simulink model "blockmodel"  (R2017b)
settings: Solver=VariableStepAuto  StartTime=0.0  StopTime=100.0  RelTol=1e-3
PreLoadFcn:
  | tic
values from neighbouring files (symbols this model uses):
  a = 1    [init.m]
  a_m = -4    [init.m]
  b = 3    [init.m]
  b_m = 4    [init.m]
  x_m_0 = 0    [init.m]
  x_p_0 = 0    [init.m]
CloseFcn:
  | toc
settings Model: Creator=q3  LastModifiedBy=q3

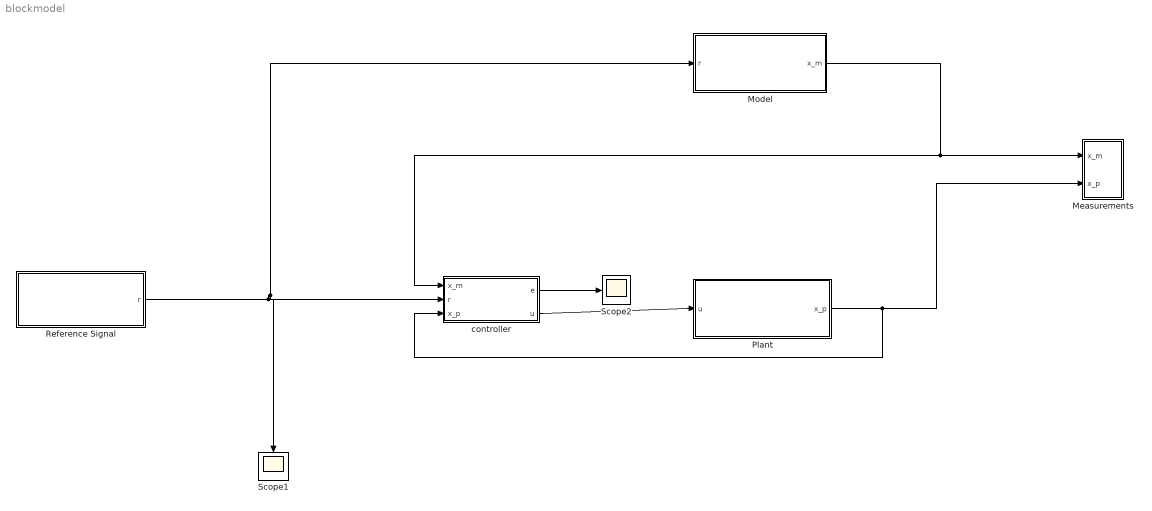
== system blockmodel ==
  Measurements : Subsystem
  Model : Subsystem
  Plant : Subsystem
  Reference Signal : Subsystem
  Scope1 : Scope
  Scope2 : Scope
  controller : Subsystem
  wires:
  controller/2(u) -> Plant/1(u)
  Model/1(x_m) -> controller/1(x_m), Measurements/1(x_m)
  Plant/1(x_p) -> controller/3(x_p), Measurements/2(x_p)
  controller/1(e) -> Scope2/1
  Reference Signal/1(r) -> Model/1(r), controller/2(r), Scope1/1

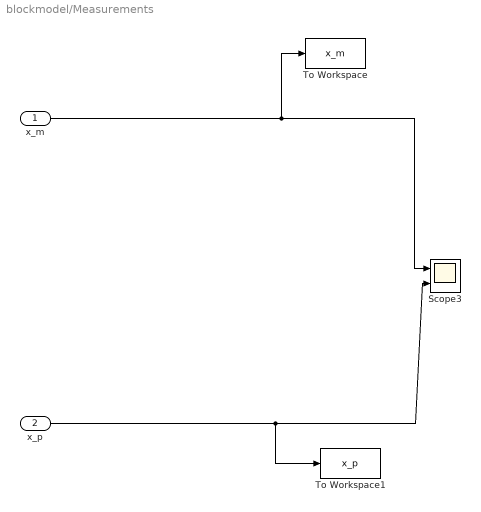
== system blockmodel/Measurements ==
  x_m : Inport
  x_p : Inport  Port=2
  Scope3 : Scope  NumInputPorts=2
  To Workspace : ToWorkspace  VariableName=x_m  SaveFormat=Timeseries  SampleTime=-1
  To Workspace1 : ToWorkspace  VariableName=x_p  SaveFormat=Timeseries  SampleTime=-1
  wires:
  x_p/1 -> Scope3/2, To Workspace1/1
  x_m/1 -> To Workspace/1, Scope3/1

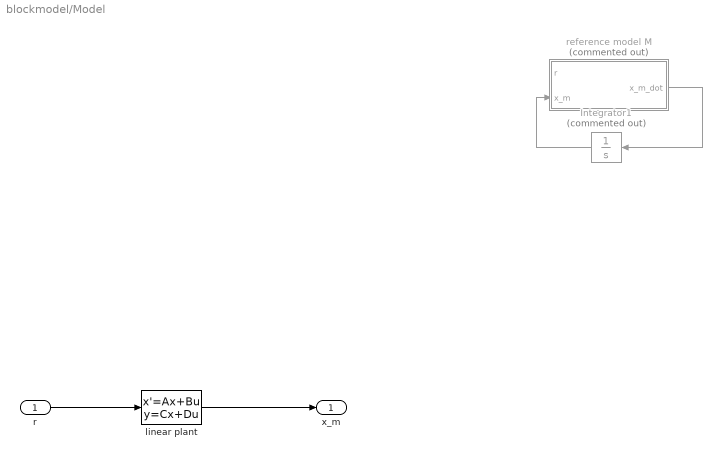
== system blockmodel/Model ==
  r : Inport
  Integrator1 : Integrator  Commented=on  InitialCondition=x_m_0
  linear plant : StateSpace  A=a_m  B=b_m  D=0  InitialCondition=x_m_0
  reference model M : MATLAB Function  Commented=on  TreatAsAtomicUnit=on
  x_m : Outport
  wires:
  reference model M/1(x_m_dot) -> Integrator1/1
  Integrator1/1 -> reference model M/2(x_m)
  r/1 -> linear plant/1
  linear plant/1 -> x_m/1

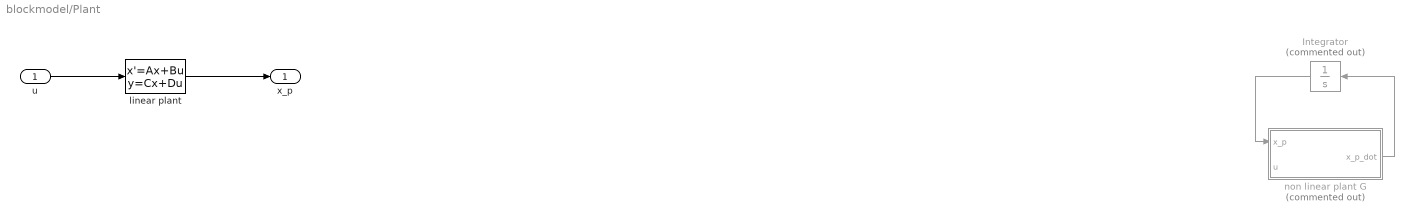
== system blockmodel/Plant ==
  u : Inport
  Integrator : Integrator  Commented=on  InitialCondition=x_p_0
  linear plant : StateSpace  A=a  B=b  D=0  InitialCondition=x_p_0
  non linear plant G : MATLAB Function  Commented=on  TreatAsAtomicUnit=on
  x_p : Outport
  wires:
  Integrator/1 -> non linear plant G/1(x_p)
  non linear plant G/1(x_p_dot) -> Integrator/1
  u/1 -> linear plant/1
  linear plant/1 -> x_p/1

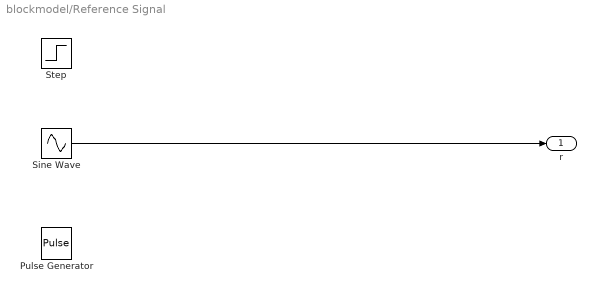
== system blockmodel/Reference Signal ==
  Pulse Generator : DiscretePulseGenerator  PulseType=Time based  Amplitude=4  PulseWidth=5
  Sine Wave : Sin  Amplitude=4  Frequency=4  SampleTime=0
  Step : Step  After=4  SampleTime=0
  r : Outport
  wires:
  Sine Wave/1 -> r/1

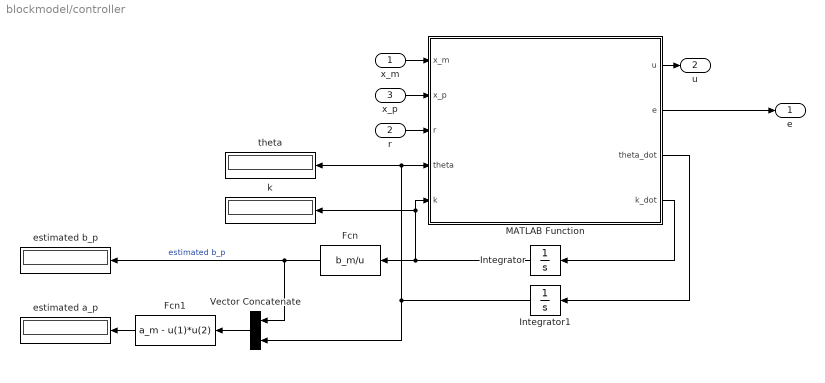
== system blockmodel/controller ==
  x_m : Inport
  r : Inport  Port=2
  x_p : Inport  Port=3
  Fcn : Fcn  Expr=b_m/u
  Fcn1 : Fcn  Expr=a_m - u(1)*u(2)
  Integrator : Integrator
  Integrator1 : Integrator
  MATLAB Function : MATLAB Function  TreatAsAtomicUnit=on
  Vector Concatenate : Concatenate
  estimated a_p : Display
  estimated b_p : Display
  k : Display
  theta : Display
  e : Outport
  u : Outport  Port=2
  wires:
  Integrator1/1 -> Vector Concatenate/2, MATLAB Function/4(theta), theta/1
  MATLAB Function/4(k_dot) -> Integrator/1
  Integrator/1 -> Fcn/1, k/1, MATLAB Function/5(k)
  MATLAB Function/2(e) -> e/1
  x_p/1 -> MATLAB Function/2(x_p)
  MATLAB Function/1(u) -> u/1
  MATLAB Function/3(theta_dot) -> Integrator1/1
  r/1 -> MATLAB Function/3(r)
  x_m/1 -> MATLAB Function/1(x_m)
  Fcn/1 -> Vector Concatenate/1, estimated b_p/1  "estimated b_p"
  Vector Concatenate/1 -> Fcn1/1
  Fcn1/1 -> estimated a_p/1

== matlab function blockmodel/Model/reference model M ==
  data: r input; x_m input; x_m_dot output
function x_m_dot = fcn(r,x_m)

% reference model equation
x_m_dot = -4*x_m + 4*r;

== matlab function blockmodel/controller/MATLAB Function ==
  data: u output; e output; x_m input; theta_dot output; x_p input; r input; k_dot output; theta input; k input
function [u,e,theta_dot,k_dot] = fcn(x_m,x_p,r,theta,k)
% adaptive gain
gamma = 2;

% error
e = x_p - x_m;

% adaptive law
theta_dot = -gamma*e*x_p;
k_dot = -gamma*e*r;

% control law
u = theta*x_p + k*r;

== matlab function blockmodel/Plant/non linear plant G ==
  data: x_p input; u input; x_p_dot output
function x_p_dot = fcn(x_p,u)

% parameter
a = 1;
b = 3;

% plant equation
x_p_dot = a*x_p + b*u;
